simulink model "self_balance_pid_discr_torquereverse_pidzn2"  (R2023b)
settings: Solver=FixedStepAuto  StartTime=0.0  StopTime=10  FixedStep=0.001  RelTol=1e-3
values from neighbouring files (symbols this model uses):
  b = 0.1    [params.mat]
  dt = 0.001    [params.mat]
  g = 9.81    [params.mat]
  I_body = 9.47333333333e-05    [params.mat]    (also in self_balance_tf.m = M_body*(l^2)/3)
  I_wheel = 1.2288e-05    [params.mat]    (also in self_balance_tf.m = M_wheel*(r^2))
  initial_angle_rad = 0    [params.mat]
  l = 0.035    [params.mat]
  M_body = 0.232    [params.mat]
  M_wheel = 0.012    [params.mat]
  r = 0.032    [params.mat]
  sat = 0.7    [params.mat]
libraries: slpidlib x1
settings Model: Creator=emamaker  LastModifiedBy=emamaker

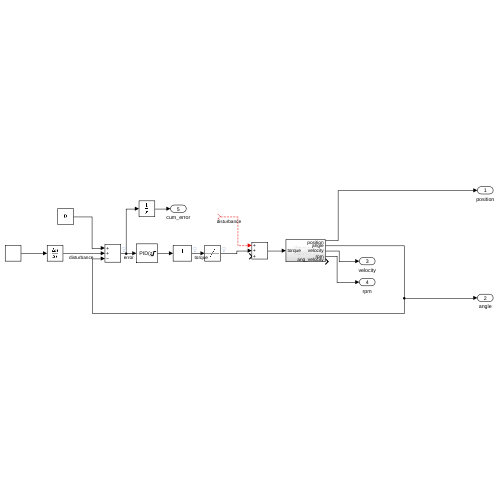
[thumbnail: Simulink's stored preview of the top-level diagram]
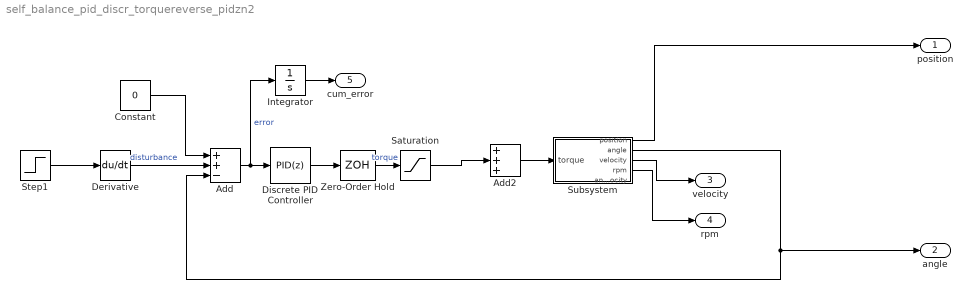
== system self_balance_pid_discr_torquereverse_pidzn2 ==
  Add : Sum  Inputs=++-
  Add2 : Sum  Inputs=+++
  Constant : Constant  Value=0
  Derivative : Derivative
  Discrete PID Controller : slpidlib/PID Controller  Controller=PID  Form=Parallel  TimeDomain=Discrete-time  UseExternalTs=off  SampleTime=dt  IntegratorMethod=Forward Euler  FilterMethod=Forward Euler  ControllerParametersSource=internal  P=6  I=0.2  UseKiTs=off  D=0.1  N=100  UseFilter=off  TunerSelectOption=Transfer Function Based (PID Tuner App)  InitialConditionSource=internal  InitialConditionForIntegrator=0  InitialConditionForFilter=0  DifferentiatorICPrevScaledInput=0  ExternalReset=none  TrackingMode=off  Kt=1  LimitOutput=on  SatLimitsSource=internal  UpperSaturationLimit=sat  LowerSaturationLimit=-sat  LinearizeAsGain=off  AntiWindupMode=clamping  Kb=1  LimitIntegrator=off  UpperIntegratorSaturationLimit=0.02  LowerIntegratorSaturationLimit=-0.02  POutMin=[]  POutMax=[]  IOutMin=[]  IOutMax=[]  DOutMin=[]  DOutMax=[]  NOutMin=[]  NOutMax=[]  SumOutMin=[]  SumOutMax=[]  SaturationOutMin=[]  SaturationOutMax=[]  PParamMin=[]  PParamMax=[]  IParamMin=[]  IParamMax=[]  DParamMin=[]  DParamMax=[]  NParamMin=[]  NParamMax=[]  KbParamMin=[]  KbParamMax=[]  KtParamMin=[]  KtParamMax=[]  KbOutMin=[]  KbOutMax=[]  KtOutMin=[]  KtOutMax=[]  IntegratorOutMin=[]  IntegratorOutMax=[]  FilterOutMin=[]  FilterOutMax=[]  SumI1OutMin=[]  SumI1OutMax=[]  SumI2OutMin=[]  SumI2OutMax=[]  SumI3OutMin=[]  SumI3OutMax=[]  SumI4OutMin=[]  SumI4OutMax=[]  SumDOutMin=[]  SumDOutMax=[]  DifferentiatorOutMin=[]  DifferentiatorOutMax=[]  FilterDiffOutCoefMin=[]  FilterDiffOutCoefMax=[]  ReciprocalOutMin=[]  ReciprocalOutMax=[]  SumDenOutMin=[]  SumDenOutMax=[]  SumNumOutMin=[]  SumNumOutMax=[]  DivideOutMin=[]  DivideOutMax=[]  UdiffTsProdOutMin=[]  UdiffTsProdOutMax=[]  NTsProdOutMin=[]  NTsProdOutMax=[]  UintegralTsProdOutMin=[]  UintegralTsProdOutMax=[]  UngainTsProdOutMin=[]  UngainTsProdOutMax=[]  ClampingZeroOutDataTypeStr=Inherit: Inherit via back propagation  ClampingZeroOutMin=[]  ClampingZeroOutMax=[]  FilterDenConstantOutDataTypeStr=Inherit: Inherit via back propagation  FilterDenConstantOutMin=[]  FilterDenConstantOutMax=[]  PCopyOutDataTypeStr=Inherit: Inherit via back propagation  PCopyOutMin=[]  PCopyOutMax=[]  NCopyOutDataTypeStr=Inherit: Inherit via back propagation  NCopyOutMin=[]  NCopyOutMax=[]  IntegratorContinuousStateAttributes=''  IntegratorStateMustResolveToSignalObject=off  IntegratorRTWStateStorageClass=Auto  FilterContinuousStateAttributes=''  FilterStateMustResolveToSignalObject=off  FilterRTWStateStorageClass=Auto  ParallelPVariant=InternalParameters  IdealPVariant=Disabled  IVariant=InternalParameters  DVariant=InternalParameters  IntegratorVariant=Discrete  SatVariant=Enabled  AWVariant=DiscClampingParallel  PCopyVariant=Disabled  TRVariant=Disabled  FdbkBlocksVariant=Forward  IdealPFdbkVariant=Disabled  SatFdbkVariant=Disabled  DerivativeFilterVariant=Differentiator  NVariant=Passthrough  NCopyVariant=Disabled_SignalSpec  FilterICVariant=InternalICsDifferentiator  IntegratorICVariant=InternalICs  ExternalResetVariant=Disabled  TRSumVariant=Passthrough  SumFdbkVariant=Disabled  SumVariant=Sum_PID  TsampFilterVariant=InternalTs  TsampNgainVariant=Passthrough  TsampIntegralVariant=Disabled_SignalSpec  ExternalSaturationOutDataTypeStr=Inherit: Same as second input
      settings: LibrarySourceBlock=simulink/Discrete/Discrete PID Controller
  Integrator : Integrator
  Saturation : Saturate  UpperLimit=sat  LowerLimit=-sat
  Step1 : Step  After=0.3  SampleTime=0.001
  Subsystem : Subsystem
  Zero-Order Hold : ZeroOrderHold  SampleTime=-1
  position : Outport
  angle : Outport  Port=2
  velocity : Outport  Port=3
  rpm : Outport  Port=4
  cum_error : Outport  Port=5
  wires:
  Add/1 -> Integrator/1, Discrete PID Controller/1  "error"
  Constant/1 -> Add/1
  Zero-Order Hold/1 -> Saturation/1  "torque"
  Subsystem/2(angle) -> Add/3, angle/1
  Subsystem/1(position) -> position/1
  Subsystem/3(velocity) -> velocity/1
  Subsystem/4(rpm) -> rpm/1
  Saturation/1 -> Add2/2
  Add2/1 -> Subsystem/1(torque)
  ? -> Add2/1  "disturbance"
  Discrete PID Controller/1 -> Zero-Order Hold/1
  Integrator/1 -> cum_error/1
  Step1/1 -> Derivative/1
  Derivative/1 -> Add/2  "disturbance"

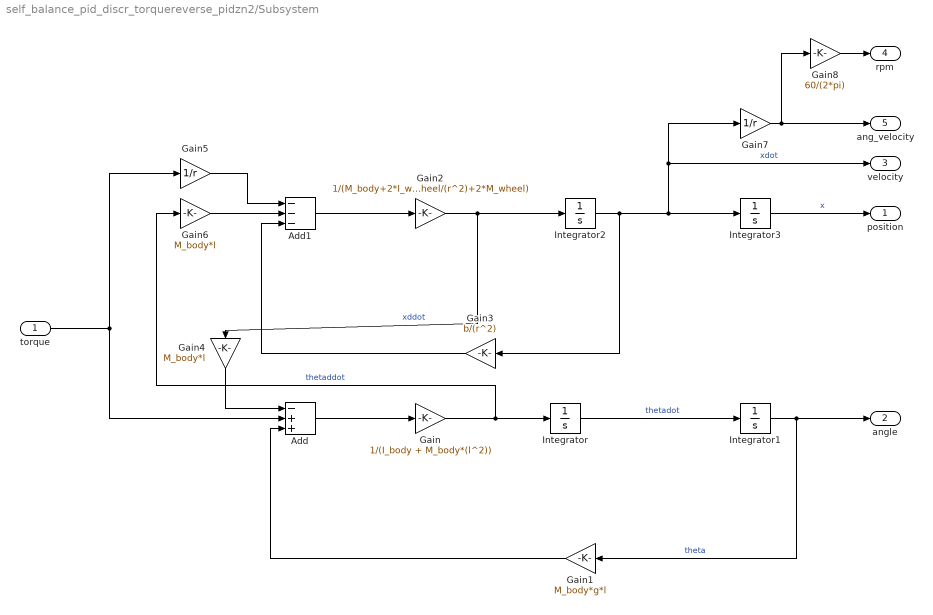
== system self_balance_pid_discr_torquereverse_pidzn2/Subsystem ==
  torque : Inport
  Add : Sum  Inputs=-++
  Add1 : Sum  Inputs=---
  Gain : Gain  Gain=1/(I_body + M_body*(l^2))
  Gain1 : Gain  Gain=M_body*g*l
  Gain2 : Gain  Gain=1/(M_body+2*I_wheel/(r^2)+2*M_wheel)
  Gain3 : Gain  Gain=b/(r^2)
  Gain4 : Gain  Gain=M_body*l
  Gain5 : Gain  Gain=1/r
  Gain6 : Gain  Gain=M_body*l
  Gain7 : Gain  Gain=1/r
  Gain8 : Gain  Gain=60/(2*pi)
  Integrator : Integrator
  Integrator1 : Integrator  InitialCondition=initial_angle_rad
  Integrator2 : Integrator
  Integrator3 : Integrator
  position : Outport
  angle : Outport  Port=2
  velocity : Outport  Port=3
  rpm : Outport  Port=4
  ang_velocity : Outport  Port=5
  wires:
  Add1/1 -> Gain2/1
  Gain5/1 -> Add1/1
  Gain1/1 -> Add/3
  Integrator2/1 -> Gain7/1, velocity/1, Integrator3/1, Gain3/1  "xdot"
  Integrator1/1 -> angle/1, Gain1/1  "theta"
  Integrator/1 -> Integrator1/1  "thetadot"
  Gain4/1 -> Add/1
  Add/1 -> Gain/1
  Integrator3/1 -> position/1  "x"
  Gain/1 -> Gain6/1, Integrator/1  "thetaddot"
  torque/1 -> Add/2, Gain5/1
  Gain3/1 -> Add1/3
  Gain2/1 -> Integrator2/1, Gain4/1  "xddot"
  Gain6/1 -> Add1/2
  Gain7/1 -> ang_velocity/1, Gain8/1
  Gain8/1 -> rpm/1
